simulink library "CoorOutlierRemoverAndFilter"  (R2018a)
settings: Solver=VariableStepAuto  StartTime=0.0  StopTime=10.0  RelTol=1e-3
undefined symbols (not defined in the file): fF, lDelay
libraries: dspfdesign x2
settings Model: Creator=Sky  LastModifiedBy=Sky

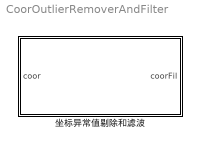
== system CoorOutlierRemoverAndFilter ==
  坐标异常值剔除和滤波 : Subsystem  mask{fF=fF}
      mask help: 根据帧率（fF）设置异常点剔除窗口大小和低通滤波器采样率。输出坐标相对输入坐标有0.5s左右的延时。

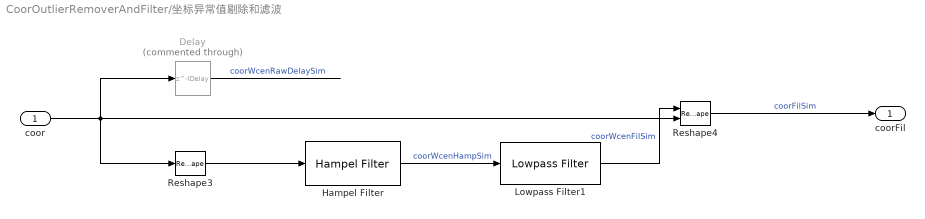
== system CoorOutlierRemoverAndFilter/坐标异常值剔除和滤波 ==
  coor : Inport
  Delay : Delay  Commented=through  DelayLength=lDelay  InitialCondition=0
  Hampel Filter : dspfdesign/Hampel Filter  WindowLength=round(fF/2)*2+1  ThresholdPort=off  Threshold=0.2  EnableIsOutlierOutput=off  SimulateUsing=Code generation
      settings: SourceProductName=DSP System Toolbox  SourceProductBaseCode=DS
  Lowpass Filter1 : dspfdesign/Lowpass Filter  FilterType=IIR  DesignForMinimumOrder=off  FilterOrder=1  PassbandFrequency=0.5  StopbandFrequency=3  PassbandRipple=0.1  StopbandAttenuation=30  InheritSampleRate=off  SampleRate=fF  SimulateUsing=Code generation  roundingMode=Floor  coeffsDataTypeStr=fixdt(1,16)
  Reshape3 : Reshape  OutputDimensionality=Row vector (2-D)
  Reshape4 : Reshape  OutputDimensionality=Derive from reference input port
  coorFil : Outport
  wires:
  Reshape3/1 -> Hampel Filter/1
  Lowpass Filter1/1 -> Reshape4/1  "coorWcenFilSim"
  Hampel Filter/1 -> Lowpass Filter1/1  "coorWcenHampSim"
  Reshape4/1 -> coorFil/1  "coorFilSim"
  coor/1 -> Reshape3/1, Reshape4/2, Delay/1
  Delay/1 -> ?  "coorWcenRawDelaySim"
